simulink model "hw1"  (R2014a)
settings: Solver=ode45  StartTime=0.0  StopTime=0.15  RelTol=1e-3
settings Model: Creator=lizhi  LastModifiedBy=lizhi

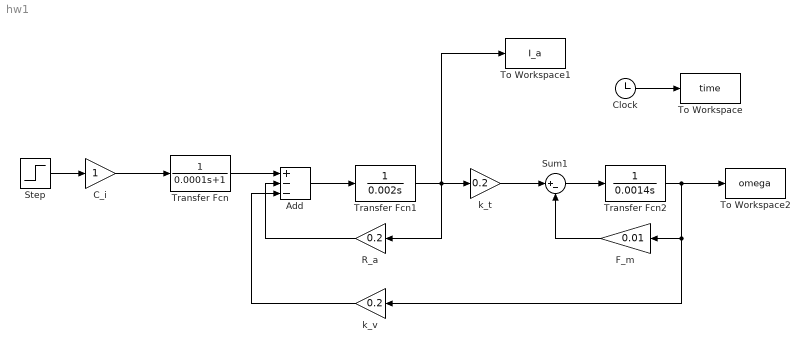
== system hw1 ==
  Add : Sum  Inputs=+--
  C_i : Gain
  Clock : Clock
  F_m : Gain  Gain=0.01
  R_a : Gain  Gain=0.2
  Step : Step  Time=0  SampleTime=0
  Sum1 : Sum  Inputs=|+-
  To Workspace : ToWorkspace  VariableName=time  SaveFormat=Timeseries  SampleTime=-1
  To Workspace1 : ToWorkspace  VariableName=I_a  SampleTime=-1
  To Workspace2 : ToWorkspace  VariableName=omega  SampleTime=-1
  Transfer Fcn : TransferFcn  Denominator=[0.0001 1]
  Transfer Fcn1 : TransferFcn  Denominator=[0.002 0]
  Transfer Fcn2 : TransferFcn  Denominator=[0.0014 0]
  k_t : Gain  Gain=0.2
  k_v : Gain  Gain=0.2
  wires:
  Step/1 -> C_i/1
  C_i/1 -> Transfer Fcn/1
  Transfer Fcn/1 -> Add/1
  Add/1 -> Transfer Fcn1/1
  Transfer Fcn1/1 -> k_t/1, To Workspace1/1, R_a/1
  k_t/1 -> Sum1/1
  Sum1/1 -> Transfer Fcn2/1
  R_a/1 -> Add/2
  F_m/1 -> Sum1/2
  k_v/1 -> Add/3
  Transfer Fcn2/1 -> To Workspace2/1, k_v/1, F_m/1
  Clock/1 -> To Workspace/1
